simulink model "sas"  (Simulink 10.1)
settings: Solver=VariableStepAuto  StartTime=0.0  StopTime=10.0  RelTol=1e-3
settings Model: Creator=jbjj  LastModifiedBy=jbjj
settings DataIOCC: SaveFormat=Dataset  ReturnWorkspaceOutputs=on
settings OptimizationCC: LifeSpan=auto
settings DebuggingCC: UnderspecifiedInitializationDetection=Simplified  MergeDetectMultiDrivingBlocksExec=error  SFUnexpectedBacktrackingDiag=error  SFNoUnconditionalDefaultTransitionDiag=error  SFExecutionAtInitializationDiag=warning  ArithmeticOperatorsInVariantConditions=error
settings HardwareCC: ProdBitPerPointer=64  ProdBitPerSizeT=64  ProdBitPerPtrDiffT=64  ProdLargestAtomicFloat=Float  ProdIntDivRoundTo=Zero  ProdEndianess=LittleEndian  ProdWordSize=64  ProdHWDeviceType=Intel->x86-64 (Windows64)
settings ModelReferenceCC: PropagateSignalLabelsOutOfModel=on
settings SFSimCC: SimUseLocalCustomCode=on  CustomCodeUndefinedFunction=FilterOut
settings RTWCC: RTWUseLocalCustomCode=on
settings CodeAppCC: StateflowObjectComments=off
settings GRTTargetCC: TargetLangStandard=C99 (ISO)  CombineOutputUpdateFcns=on  GRTInterface=off
settings ConfigComp: CovMetricSettings=dwe  CovHtmlReporting=off  CovSaveCumulativeToWorkspaceVar=off  CovSaveSingleToWorkspaceVar=off  CovExternalEMLEnable=on

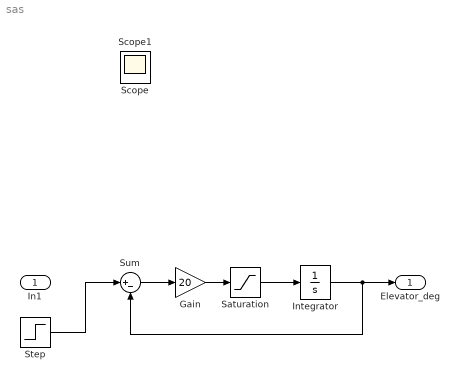
== system sas ==
  In1 : Inport
  Gain : Gain  Gain=20
  Integrator : Integrator  LimitOutput=on  UpperSaturationLimit=15  LowerSaturationLimit=-25
  Saturation : Saturate  UpperLimit=40  LowerLimit=-40
  Step : Step  SampleTime=0
  Sum : Sum  Inputs=|+-
  Elevator_deg : Outport
  Scope : Scope
  Scope1 : Scope
  wires:
  Integrator/1 -> Sum/2, Elevator_deg/1
  Saturation/1 -> Integrator/1
  Sum/1 -> Gain/1
  Step/1 -> Sum/1
  Gain/1 -> Saturation/1
